simulink model "sbw_actuator_new260308_forCar"  (R2025b)
settings: Solver=ode5  StartTime=0.0  StopTime=10  FixedStep=0.0001  RelTol=1e-3
InitFcn:
  | %% 转向执行总成参数
  | % 电机输出轴
  | I_sam = 0.02;                 % kg·m^2
  | B_sam = 0.002 * 180/pi;                 % N·m·s/rad
  | K_fsam = 0.2;                  % N·m
  | 
  | % 齿条
  | M_sr = 32.47;                     % kg
  | B_sr = 5500;                     % N·s/m
  | K_fsr =300;                     % N
  | 
  | % 结构参数
  | k_bm = 17600;                     % N·m/rad
  | i_bs =  111.7011;         % rad/m
libraries: Solver_SF x1
settings Model: Creator=23649  LastModifiedBy=23649

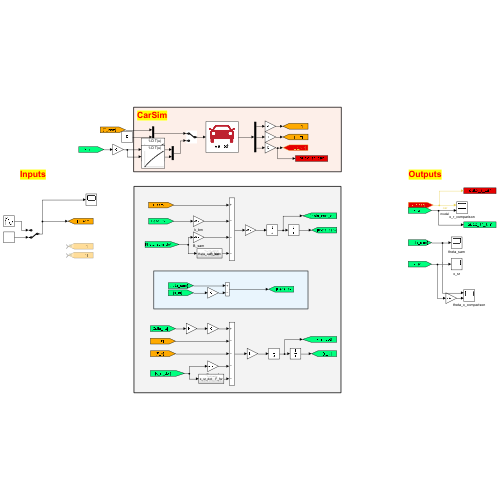
[thumbnail: Simulink's stored preview of the top-level diagram]
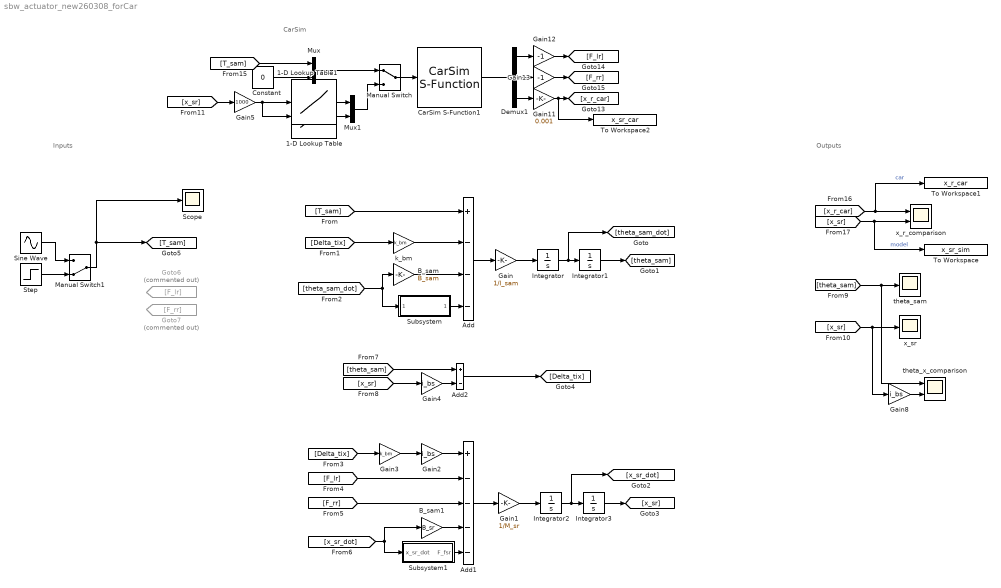
== system sbw_actuator_new260308_forCar ==
  note: CarSim
  note: Inputs
  note: Outputs
  1-D Lookup Table : Lookup_n-D  NumberOfTableDimensions=1  BreakpointsForDimension1=[-90;-89.099999999999994;-88.200000000000003;-87.299999999999997;-86.400000000000006;-85.5;-84.599999999999994;-83.700000000000003;-82.799999999999997;-81.900000000000006;-81;-80.099999999999994;-79.200000000000003;-78.299999999999997;-77.400000000000006;-76.5;-75.599999999999994;-74.700000000000003;-73.799999999999997;-72.900000000000006;-72;-71.099999999999994;-70.200000000000003;-69.299999999999997;-68.400000000000006;-67.5;-66.599999999999994;-65.700000000000003;-64.799999999999997;-63.899999999999999;-63;-62.100000000000001;-61.200000000000003;-60.299999999999997;-59.399999999999999;-58.5;-57.600000000000001;-56.700000000000003;-55.799999999999997;-54.899999999999999;-54;-53.100000000000001;-52.200000000000003;-51.299999999999997;-50.399999999999999;-49.5;-48.600000000000001;-47.700000000000003;-46.799999999999997;-45.899999999999999;-45;-44.100000000000001;-43.200000000000003;-42.299999999999997;-41.399999999999999;-40.5;-39.600000000000001;-38.700000000000003;-37.799999999999997;-36.899999999999999;-36;-35.100000000000001;-34.200000000000003;-33.299999999999997;-32.399999999999999;-31.5;-30.600000000000001;-29.699999999999999;-28.800000000000001;-27.899999999999999;-27;-26.100000000000001;-25.199999999999999;-24.300000000000001;-23.399999999999999;-22.5;-21.600000000000001;-20.699999999999999;-19.800000000000001;-18.899999999999999;-18;-17.100000000000001;-16.199999999999999;-15.300000000000001;-14.4;-13.5;-12.6;-11.699999999999999;-10.800000000000001;-9.9000000000000004;-9;-8.0999999999999996;-7.2000000000000002;-6.2999999999999998;-5.4000000000000004;-4.5;-3.6000000000000001;-2.7000000000000002;-1.8;-0.90000000000000002;0;0.90000000000000002;1.8;2.7000000000000002;3.6000000000000001;4.5;5.4000000000000004;6.2999999999999998;7.2000000000000002;8.0999999999999996;9;9.9000000000000004;10.800000000000001;11.699999999999999;12.6;13.5;14.4;15.300000000000001;16.199999999999999;17.100000000000001;18;18.899999999999999;19.800000000000001;20.699999999999999;21.600000000000001;22.5;23.399999999999999;24.300000000000001;25.199999999999999;26.100000000000001;27;27.899999999999999;28.800000000000001;29.699999999999999;30.600000000000001;31.5;32.399999999999999;33.299999999999997;34.200000000000003;35.100000000000001;36;36.899999999999999;37.799999999999997;38.700000000000003;39.600000000000001;40.5;41.399999999999999;42.299999999999997;43.200000000000003;44.100000000000001;45;45.899999999999999;46.799999999999997;47.700000000000003;48.600000000000001;49.5;50.399999999999999;51.299999999999997;52.200000000000003;53.100000000000001;54;54.899999999999999;55.799999999999997;56.700000000000003;57.600000000000001;58.5;59.399999999999999;60.299999999999997;61.200000000000003;62.100000000000001;63;63.899999999999999;64.799999999999997;65.700000000000003;66.599999999999994;67.5;68.400000000000006;69.299999999999997;70.200000000000003;71.099999999999994;72;72.900000000000006;73.799999999999997;74.700000000000003;75.599999999999994;76.5;77.400000000000006;78.299999999999997;79.200000000000003;80.099999999999994;81;81.900000000000006;82.799999999999997;83.700000000000003;84.599999999999994;85.5;86.400000000000006;87.299999999999997;88.200000000000003;89.099999999999994;90]  Table=[-44.966654550000001;-44.37881522;-43.794882540000003;-43.214803580000002;-42.638527179999997;-42.066003889999998;-41.497185799999997;-40.932026489999998;-40.370480909999998;-39.812505280000003;-39.258057030000003;-38.707094730000001;-38.159577970000001;-37.615467359999997;-37.074724420000003;-36.537311539999997;-36.003191940000001;-35.472329600000002;-34.944689220000001;-34.420236180000003;-33.898936499999998;-33.3807568;-32.865664279999997;-32.353626650000002;-31.844612160000001;-31.338589509999998;-30.835527859999999;-30.335396809999999;-29.838166350000002;-29.343806860000001;-28.852289079999998;-28.363584110000001;-27.87766337;-27.394498590000001;-26.914061799999999;-26.436325329999999;-25.961261759999999;-25.48884395;-25.019044990000001;-24.551838239999999;-24.087197249999999;-23.625095810000001;-23.165507940000001;-22.708407829999999;-22.253769890000001;-21.801568710000002;-21.351779059999998;-20.904375909999999;-20.459334370000001;-20.016629739999999;-19.57623748;-19.138133190000001;-18.70229265;-18.268691759999999;-17.837306590000001;-17.40811334;-16.981088339999999;-16.556208089999998;-16.13344918;-15.712788339999999;-15.294202459999999;-14.877668509999999;-14.4631636;-14.05066497;-13.64014997;-13.23159605;-12.82498079;-12.420281879999999;-12.01747711;-11.61654439;-11.217461719999999;-10.820207229999999;-10.42475911;-10.03109568;-9.6391953620000006;-9.2490366559999995;-8.8605981679999992;-8.4738585919999991;-8.0887967179999993;-7.7053914209999999;-7.3236216680000004;-6.9434665100000004;-6.5649050830000002;-6.1879166059999999;-5.8124803780000001;-5.4385757779999997;-5.066182263;-4.6952793650000002;-4.3258466880000004;-3.9578639099999999;-3.591310778;-3.226167105;-2.862412773;-2.5000277259999999;-2.138991968;-1.779285564;-1.4208886359999999;-1.0637813620000001;-0.70794396999999998;-0.35335674;0;0.35214587800000002;0.70310047799999997;1.0528833440000001;1.4015139830000001;1.749011868;2.0953964369999998;2.4406871020000001;2.7849032469999999;3.1280642329999999;3.4701894009999998;3.811298077;4.1514095690000001;4.4905431790000003;4.8287181979999998;5.1659539179999996;5.5022696260000004;5.8376846179999999;6.172218193;6.5058896639999997;6.8387183599999997;7.170723626;7.5019248359999997;7.8323413879999997;8.1619927140000001;8.4908982829999999;8.8190776060000005;9.1465502399999998;9.4733357950000006;9.7994539379999992;10.12492439;10.44976696;10.77400151;11.09764799;11.420726419999999;11.74325694;12.06525976;12.38675522;12.70776373;13.028305870000001;13.3484023;13.66807384;13.98734144;14.30622619;14.624749339999999;14.94293233;15.260796729999999;15.57836432;15.89565707;16.212697160000001;16.529506940000001;16.846109040000002;17.162526289999999;17.47878176;17.794898799999999;18.110900999999998;18.426812269999999;18.742656780000001;19.058459020000001;19.374243809999999;19.690036289999998;20.00586199;20.321746770000001;20.637716900000001;20.953799050000001;21.270020299999999;21.586408200000001;21.902990729999999;22.219796389999999;22.536854160000001;22.854193559999999;23.171844650000001;23.4898381;23.80820516;24.126977709999998;24.446188329999998;24.765870249999999;25.086057459999999;25.406784699999999;25.728087510000002;26.050002259999999;26.372566209999999;26.695817529999999;27.019795349999999;27.344539829999999;27.67009217;27.9964947;28.32379091;28.652025519999999;28.98124456;29.311495409999999;29.642826880000001;29.975289279999998;30.308934529999998;30.643816210000001;30.979989669999998;31.317512130000001;31.65644275;31.996842820000001;32.33877579;32.682307459999997]  InternalRulePriority=Speed  RndMeth=Simplest
  1-D Lookup Table1 : Lookup_n-D  NumberOfTableDimensions=1  BreakpointsForDimension1=[-90;-89.099999999999994;-88.200000000000003;-87.299999999999997;-86.400000000000006;-85.5;-84.599999999999994;-83.700000000000003;-82.799999999999997;-81.900000000000006;-81;-80.099999999999994;-79.200000000000003;-78.299999999999997;-77.400000000000006;-76.5;-75.599999999999994;-74.700000000000003;-73.799999999999997;-72.900000000000006;-72;-71.099999999999994;-70.200000000000003;-69.299999999999997;-68.400000000000006;-67.5;-66.599999999999994;-65.700000000000003;-64.799999999999997;-63.899999999999999;-63;-62.100000000000001;-61.200000000000003;-60.299999999999997;-59.399999999999999;-58.5;-57.600000000000001;-56.700000000000003;-55.799999999999997;-54.899999999999999;-54;-53.100000000000001;-52.200000000000003;-51.299999999999997;-50.399999999999999;-49.5;-48.600000000000001;-47.700000000000003;-46.799999999999997;-45.899999999999999;-45;-44.100000000000001;-43.200000000000003;-42.299999999999997;-41.399999999999999;-40.5;-39.600000000000001;-38.700000000000003;-37.799999999999997;-36.899999999999999;-36;-35.100000000000001;-34.200000000000003;-33.299999999999997;-32.399999999999999;-31.5;-30.600000000000001;-29.699999999999999;-28.800000000000001;-27.899999999999999;-27;-26.100000000000001;-25.199999999999999;-24.300000000000001;-23.399999999999999;-22.5;-21.600000000000001;-20.699999999999999;-19.800000000000001;-18.899999999999999;-18;-17.100000000000001;-16.199999999999999;-15.300000000000001;-14.4;-13.5;-12.6;-11.699999999999999;-10.800000000000001;-9.9000000000000004;-9;-8.0999999999999996;-7.2000000000000002;-6.2999999999999998;-5.4000000000000004;-4.5;-3.6000000000000001;-2.7000000000000002;-1.8;-0.90000000000000002;0;0.90000000000000002;1.8;2.7000000000000002;3.6000000000000001;4.5;5.4000000000000004;6.2999999999999998;7.2000000000000002;8.0999999999999996;9;9.9000000000000004;10.800000000000001;11.699999999999999;12.6;13.5;14.4;15.300000000000001;16.199999999999999;17.100000000000001;18;18.899999999999999;19.800000000000001;20.699999999999999;21.600000000000001;22.5;23.399999999999999;24.300000000000001;25.199999999999999;26.100000000000001;27;27.899999999999999;28.800000000000001;29.699999999999999;30.600000000000001;31.5;32.399999999999999;33.299999999999997;34.200000000000003;35.100000000000001;36;36.899999999999999;37.799999999999997;38.700000000000003;39.600000000000001;40.5;41.399999999999999;42.299999999999997;43.200000000000003;44.100000000000001;45;45.899999999999999;46.799999999999997;47.700000000000003;48.600000000000001;49.5;50.399999999999999;51.299999999999997;52.200000000000003;53.100000000000001;54;54.899999999999999;55.799999999999997;56.700000000000003;57.600000000000001;58.5;59.399999999999999;60.299999999999997;61.200000000000003;62.100000000000001;63;63.899999999999999;64.799999999999997;65.700000000000003;66.599999999999994;67.5;68.400000000000006;69.299999999999997;70.200000000000003;71.099999999999994;72;72.900000000000006;73.799999999999997;74.700000000000003;75.599999999999994;76.5;77.400000000000006;78.299999999999997;79.200000000000003;80.099999999999994;81;81.900000000000006;82.799999999999997;83.700000000000003;84.599999999999994;85.5;86.400000000000006;87.299999999999997;88.200000000000003;89.099999999999994;90]  Table=[-44.966654550000001;-44.37881522;-43.794882540000003;-43.214803580000002;-42.638527179999997;-42.066003889999998;-41.497185799999997;-40.932026489999998;-40.370480909999998;-39.812505280000003;-39.258057030000003;-38.707094730000001;-38.159577970000001;-37.615467359999997;-37.074724420000003;-36.537311539999997;-36.003191940000001;-35.472329600000002;-34.944689220000001;-34.420236180000003;-33.898936499999998;-33.3807568;-32.865664279999997;-32.353626650000002;-31.844612160000001;-31.338589509999998;-30.835527859999999;-30.335396809999999;-29.838166350000002;-29.343806860000001;-28.852289079999998;-28.363584110000001;-27.87766337;-27.394498590000001;-26.914061799999999;-26.436325329999999;-25.961261759999999;-25.48884395;-25.019044990000001;-24.551838239999999;-24.087197249999999;-23.625095810000001;-23.165507940000001;-22.708407829999999;-22.253769890000001;-21.801568710000002;-21.351779059999998;-20.904375909999999;-20.459334370000001;-20.016629739999999;-19.57623748;-19.138133190000001;-18.70229265;-18.268691759999999;-17.837306590000001;-17.40811334;-16.981088339999999;-16.556208089999998;-16.13344918;-15.712788339999999;-15.294202459999999;-14.877668509999999;-14.4631636;-14.05066497;-13.64014997;-13.23159605;-12.82498079;-12.420281879999999;-12.01747711;-11.61654439;-11.217461719999999;-10.820207229999999;-10.42475911;-10.03109568;-9.6391953620000006;-9.2490366559999995;-8.8605981679999992;-8.4738585919999991;-8.0887967179999993;-7.7053914209999999;-7.3236216680000004;-6.9434665100000004;-6.5649050830000002;-6.1879166059999999;-5.8124803780000001;-5.4385757779999997;-5.066182263;-4.6952793650000002;-4.3258466880000004;-3.9578639099999999;-3.591310778;-3.226167105;-2.862412773;-2.5000277259999999;-2.138991968;-1.779285564;-1.4208886359999999;-1.0637813620000001;-0.70794396999999998;-0.35335674;0;0.35214587800000002;0.70310047799999997;1.0528833440000001;1.4015139830000001;1.749011868;2.0953964369999998;2.4406871020000001;2.7849032469999999;3.1280642329999999;3.4701894009999998;3.811298077;4.1514095690000001;4.4905431790000003;4.8287181979999998;5.1659539179999996;5.5022696260000004;5.8376846179999999;6.172218193;6.5058896639999997;6.8387183599999997;7.170723626;7.5019248359999997;7.8323413879999997;8.1619927140000001;8.4908982829999999;8.8190776060000005;9.1465502399999998;9.4733357950000006;9.7994539379999992;10.12492439;10.44976696;10.77400151;11.09764799;11.420726419999999;11.74325694;12.06525976;12.38675522;12.70776373;13.028305870000001;13.3484023;13.66807384;13.98734144;14.30622619;14.624749339999999;14.94293233;15.260796729999999;15.57836432;15.89565707;16.212697160000001;16.529506940000001;16.846109040000002;17.162526289999999;17.47878176;17.794898799999999;18.110900999999998;18.426812269999999;18.742656780000001;19.058459020000001;19.374243809999999;19.690036289999998;20.00586199;20.321746770000001;20.637716900000001;20.953799050000001;21.270020299999999;21.586408200000001;21.902990729999999;22.219796389999999;22.536854160000001;22.854193559999999;23.171844650000001;23.4898381;23.80820516;24.126977709999998;24.446188329999998;24.765870249999999;25.086057459999999;25.406784699999999;25.728087510000002;26.050002259999999;26.372566209999999;26.695817529999999;27.019795349999999;27.344539829999999;27.67009217;27.9964947;28.32379091;28.652025519999999;28.98124456;29.311495409999999;29.642826880000001;29.975289279999998;30.308934529999998;30.643816210000001;30.979989669999998;31.317512130000001;31.65644275;31.996842820000001;32.33877579;32.682307459999997]  InternalRulePriority=Speed  RndMeth=Simplest
  Add : Sum  Inputs=+---
  Add1 : Sum  Inputs=+----
  Add2 : Sum  Inputs=+-
  B_sam : Gain  Gain=B_sam
  B_sam1 : Gain  Gain=B_sr
  CarSim S-Function1 : Solver_SF/CarSim S-Function  Priority=1  SIMFILE=simfile.sim  Run_RTs=off  vs_state_ind=Run  StopMode_ind=Vehicle Model
  Constant : Constant  Value=0
  Demux1 : Demux  Outputs=3
  Gain : Gain  Gain=1/I_sam
  Gain1 : Gain  Gain=1/M_sr
  Gain11 : Gain  Gain=0.001
  Gain12 : Gain  Gain=-1
  Gain13 : Gain  Gain=-1
  Gain2 : Gain  Gain=i_bs
  Gain3 : Gain  Gain=k_bm
  Gain4 : Gain  Gain=i_bs
  Gain5 : Gain  Gain=1000
  Gain8 : Gain  Gain=i_bs
  Goto6 : Goto  Commented=on  GotoTag=F_lr
  Goto7 : Goto  Commented=on  GotoTag=F_rr
  Integrator{,1..3} (4 alike) : Integrator
  Manual Switch : ManualSwitch
  Manual Switch1 : ManualSwitch  CurrentSetting=0
  Mux : Mux  Inputs=2
  Mux1 : Mux  Inputs=2
  Scope : Scope
      settings: ActiveDisplayYMinimum=-1.1062993060853035  ActiveDisplayYMaximum=1.1612743899833331  DataLoggingVariableName=ScopeData3
  Sine Wave : Sin  Amplitude=10  SampleTime=0
  Step : Step  Time=3  After=15  SampleTime=0
  Subsystem : Subsystem
  Subsystem1 : Subsystem
  To Workspace : ToWorkspace  VariableName=x_sr_sim  SampleTime=-1
  To Workspace1 : ToWorkspace  VariableName=x_r_car  SampleTime=-1
  To Workspace2 : ToWorkspace  VariableName=x_sr_car  SampleTime=-1
  k_bm : Gain  Gain=k_bm
  theta_sam : Scope
      settings: ActiveDisplayYMinimum=-70.932509033665454  ActiveDisplayYMaximum=638.39257783018445
  theta_x_comparison : Scope  NumInputPorts=2
      settings: ActiveDisplayYMinimum=-0.2821878575554751  ActiveDisplayYMaximum=0.29784467862323083  DataLoggingVariableName=ScopeData2
  x_r_comparison : Scope  NumInputPorts=2
      settings: ActiveDisplayYMinimum=-0.0021359873119448617  ActiveDisplayYMaximum=0.002204732698880189  DataLoggingVariableName=ScopeData5
  x_sr : Scope
      settings: ActiveDisplayYMinimum=-1  ActiveDisplayYMaximum=1
  wires:
  Add/1 -> Gain/1
  Gain/1 -> Integrator/1
  [T_sam] -> Add/1
  k_bm/1 -> Add/2
  [Delta_tix] -> k_bm/1
  B_sam/1 -> Add/3
  [theta_sam_dot] -> B_sam/1, Subsystem/1(theta_sam_dot)
  Subsystem/1(F_fsam) -> Add/4
  Integrator/1 -> Integrator1/1, [theta_sam_dot]
  Integrator1/1 -> [theta_sam]
  Integrator3/1 -> [x_sr]
  Integrator2/1 -> Integrator3/1, [x_sr_dot]
  Gain1/1 -> Integrator2/1
  Add1/1 -> Gain1/1
  [Delta_tix] -> Gain3/1
  Gain2/1 -> Add1/1
  Gain3/1 -> Gain2/1
  [F_lr] -> Add1/2
  [F_rr] -> Add1/3
  B_sam1/1 -> Add1/4
  [x_sr_dot] -> B_sam1/1, Subsystem1/1(x_sr_dot)
  Subsystem1/1(F_fsr) -> Add1/5
  Add2/1 -> [Delta_tix]
  [x_sr] -> Gain4/1
  [theta_sam] -> Add2/1
  Gain4/1 -> Add2/2
  Manual Switch1/1 -> [T_sam], Scope/1
  [theta_sam] -> theta_sam/1, theta_x_comparison/1
  Gain8/1 -> theta_x_comparison/2
  [x_sr] -> Gain8/1, x_sr/1
  CarSim S-Function1/1 -> Demux1/1
  Demux1/3 -> Gain11/1
  Demux1/2 -> Gain13/1
  Demux1/1 -> Gain12/1
  Gain11/1 -> To Workspace2/1, [x_r_car]
  [x_r_car] -> To Workspace1/1, x_r_comparison/1  "car"
  [x_sr] -> To Workspace/1, x_r_comparison/2  "model"
  Gain12/1 -> [F_lr]
  Gain13/1 -> [F_rr]
  Manual Switch/1 -> CarSim S-Function1/1
  [T_sam] -> Mux/1
  [x_sr] -> Gain5/1
  Mux1/1 -> Manual Switch/2
  Mux/1 -> Manual Switch/1
  1-D Lookup Table1/1 -> Mux1/1
  1-D Lookup Table/1 -> Mux1/2
  Constant/1 -> Mux/2
  Gain5/1 -> 1-D Lookup Table/1, 1-D Lookup Table1/1
  Sine Wave/1 -> Manual Switch1/1
  Step/1 -> Manual Switch1/2

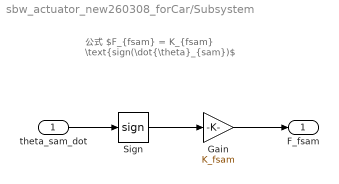
== system sbw_actuator_new260308_forCar/Subsystem ==
  note: 公式 $F_{fsam} = K_{fsam} \text{sign(\dot{\theta}_{sam})$
  theta_sam_dot : Inport
  Gain : Gain  Gain=K_fsam
  Sign : Signum
  F_fsam : Outport
  wires:
  theta_sam_dot/1 -> Sign/1
  Gain/1 -> F_fsam/1
  Sign/1 -> Gain/1

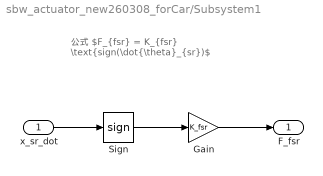
== system sbw_actuator_new260308_forCar/Subsystem1 ==
  note: 公式 $F_{fsr} = K_{fsr} \text{sign(\dot{\theta}_{sr})$
  x_sr_dot : Inport
  Gain : Gain  Gain=K_fsr
  Sign : Signum
  F_fsr : Outport
  wires:
  x_sr_dot/1 -> Sign/1
  Gain/1 -> F_fsr/1
  Sign/1 -> Gain/1
